simulink library "Library_ASK"  (R2018b)
settings: Solver=VariableStepAuto  StartTime=0.0  StopTime=10.0  RelTol=1e-3  EnableMultiTasking=on
undefined symbols (not defined in the file): akt_2GTR_az_HA, akt_2GTR_az_VA, akt_2GTR_rn_HA, akt_2GTR_rn_VA, akt_GTR_az_HA, akt_GTR_az_VA, akt_GTR_rn_HA, akt_GTR_rn_VA, alpha, b_zahn, beta_b, breakpointset, choose_ulg, DiscIntNeverNeededParam, eps_1, eps_2, eps_alpha, eta_aa, eta_Kegel_max, Fx_LSD_max, Fx_mUELG_max, i_DF, i_Kegelrad_OD, i_TRM_G1_HA, i_TRM_G1_VA, i_TRM_G2_HA, i_TRM_G2_VA, i_TRM_HA, i_TRM_Stufe_1_HA, i_TRM_Stufe_1_VA, i_TRM_Stufe_2_HA, i_TRM_Stufe_2_VA, i_TRM_VA, M_Cl_LSD_max, M_Cl_mUELG_max, M_EM_max, M_Kupplung_mUELG_Schlepp, mu_cl_LSD, mu_cl_mUELG, n_EM_max, n_Stufen_TRM_HA, n_Stufen_TRM_VA, ndyn_oil, nreib_LSD, nreib_mUELG, par_MDT, par_VEH, Ra, rm_LSD, rm_mUELG, select_Traktion_split, stepsize, wkg_Diff_mUELG, wkg_GTR, X_L, z_atts, z_ayc, z_ayc_lr, z_ayc_rl
libraries: simulink x23, $bdroot x6
(part 3 of 4)

== system Library_ASK/Mehrstufiges und mehrgängiges Getriebe/Subsystem ==
  WKG : Inport
  Inputleistung : Inport  Port=2
  Abs : Abs
  Add : Sum  Inputs=+-
  Constant : Constant
  Product5 : Product
  "W -> kW" : Gain  Gain=0.001
  Verlustleistung [kW] : Outport
  wires:
  Constant/1 -> Add/1
  Inputleistung/1 -> Product5/2
  Add/1 -> Product5/1
  Abs/1 -> "W -> kW"/1
  Product5/1 -> Abs/1
  "W -> kW"/1 -> Verlustleistung [kW]/1
  WKG/1 -> Add/2

== system Library_ASK/Momentenrückführung az HA/Fall Eingängiges Getriebe ==
  Radwunschmoment : Inport
  eta_HA : Inport  Port=2
  Enable : EnablePort
  Constant : Constant  Value=i_TRM_HA
  Divide2 : Product  Inputs=*//
  Motorwunschmoment : Outport
  wires:
  Radwunschmoment/1 -> Divide2/1
  Constant/1 -> Divide2/2
  Divide2/1 -> Motorwunschmoment/1
  eta_HA/1 -> Divide2/3

== system Library_ASK/Momentenrückführung az HA/Fall zweigängiges Getriebe ==
  note: auf diese Weise wird die Goto/From - Rückführung aus dem EM -Block überflüssig
  Radwunschmoment : Inport
  Mittlere Raddrehzahl : Inport  Port=2
  eta_HA : Inport  Port=3
  Enable : EnablePort
  Constant : Constant  Value=i_TRM_G1_HA
  Constant1 : Constant  Value=i_TRM_G2_HA
  Constant2 : Constant  Value=n_EM_max
  Divide1 : Product  Inputs=*//
  MATLAB Function : MATLAB Function  TreatAsAtomicUnit=on
  Product : Product
  Motorwunschmoment : Outport
  wires:
  Product/1 -> MATLAB Function/1(n_EM)
  Mittlere Raddrehzahl/1 -> Product/1
  Divide1/1 -> Motorwunschmoment/1
  Constant/1 -> MATLAB Function/3(i_TRM_G1), Product/2
  Radwunschmoment/1 -> Divide1/1
  MATLAB Function/1(i_TRM) -> Divide1/2
  Constant1/1 -> MATLAB Function/4(i_TRM_G2)
  Constant2/1 -> MATLAB Function/2(n_EM_max)
  eta_HA/1 -> Divide1/3

== system Library_ASK/Momentenrückführung az VA/Fall Eingängiges Getriebe ==
  Radwunschmoment : Inport
  eta_VA : Inport  Port=2
  Enable : EnablePort
  Constant : Constant  Value=i_TRM_VA
  Divide2 : Product  Inputs=*//
  Motorwunschmoment : Outport
  wires:
  Divide2/1 -> Motorwunschmoment/1
  Constant/1 -> Divide2/2
  Radwunschmoment/1 -> Divide2/1
  eta_VA/1 -> Divide2/3

== system Library_ASK/Momentenrückführung az VA/Fall zweigängiges Getriebe ==
  note: auf diese Weise wird die Goto/From - Rückführung aus dem EM -Block überflüssig
  Radwunschmoment : Inport
  Mittlere Raddrehzahl : Inport  Port=2
  eta_VA : Inport  Port=3
  Enable : EnablePort
  Constant : Constant  Value=i_TRM_G1_VA
  Constant1 : Constant  Value=i_TRM_G2_VA
  Constant2 : Constant  Value=n_EM_max
  Divide1 : Product  Inputs=*//
  MATLAB Function : MATLAB Function  TreatAsAtomicUnit=on
  Product : Product
  Motorwunschmoment : Outport
  wires:
  Constant2/1 -> MATLAB Function/2(n_EM_max)
  Constant1/1 -> MATLAB Function/4(i_TRM_G2)
  MATLAB Function/1(i_TRM) -> Divide1/2
  Radwunschmoment/1 -> Divide1/1
  Constant/1 -> Product/2, MATLAB Function/3(i_TRM_G1)
  Divide1/1 -> Motorwunschmoment/1
  Mittlere Raddrehzahl/1 -> Product/1
  Product/1 -> MATLAB Function/1(n_EM)
  eta_VA/1 -> Divide1/3

== system Library_ASK/Momentenrückführung rn HA/Fall Eingängiges Getriebe ==
  Radwunschmoment : Inport
  eta_HA : Inport  Port=2
  Enable : EnablePort
  Constant : Constant  Value=i_TRM_HA
  Divide2 : Product  Inputs=*//
  Motorwunschmoment : Outport
  wires:
  Divide2/1 -> Motorwunschmoment/1
  Constant/1 -> Divide2/2
  Radwunschmoment/1 -> Divide2/1
  eta_HA/1 -> Divide2/3

== system Library_ASK/Momentenrückführung rn HA/Fall zweigängiges Getriebe ==
  note: auf diese Weise wird die Goto/From - Rückführung aus dem EM -Block überflüssig
  Radwunschmoment : Inport
  Raddrehzahl : Inport  Port=2
  eta_HA : Inport  Port=3
  Enable : EnablePort
  Constant : Constant  Value=i_TRM_G1_HA
  Constant1 : Constant  Value=i_TRM_G2_HA
  Constant2 : Constant  Value=n_EM_max
  Demux : Demux  Outputs=2
  Divide1 : Product  Inputs=*//
  MATLAB Function : MATLAB Function  TreatAsAtomicUnit=on
  MATLAB Function1 : MATLAB Function  TreatAsAtomicUnit=on
  Mux : Mux  Inputs=2
  Product : Product
  Motorwunschmoment : Outport
  wires:
  MATLAB Function1/1(i_TRM) -> Mux/2
  MATLAB Function/1(i_TRM) -> Mux/1
  Mux/1 -> Divide1/2
  Demux/2 -> MATLAB Function1/1(n_EM)  "Linkes Rad"
  Demux/1 -> MATLAB Function/1(n_EM)  "Rechtes Rad"
  Constant2/1 -> MATLAB Function/2(n_EM_max), MATLAB Function1/2(n_EM_max)
  Constant1/1 -> MATLAB Function/4(i_TRM_G2), MATLAB Function1/4(i_TRM_G2)
  Radwunschmoment/1 -> Divide1/1
  Constant/1 -> Product/2, MATLAB Function/3(i_TRM_G1), MATLAB Function1/3(i_TRM_G1)
  Divide1/1 -> Motorwunschmoment/1
  Raddrehzahl/1 -> Product/1
  Product/1 -> Demux/1
  eta_HA/1 -> Divide1/3

== system Library_ASK/Momentenrückführung rn VA/Fall Eingängiges Getriebe ==
  Radwunschmoment : Inport
  eta_VA : Inport  Port=2
  Enable : EnablePort
  Constant : Constant  Value=i_TRM_VA
  Divide2 : Product  Inputs=*//
  Motorwunschmoment : Outport
  wires:
  Radwunschmoment/1 -> Divide2/1
  Constant/1 -> Divide2/2
  Divide2/1 -> Motorwunschmoment/1
  eta_VA/1 -> Divide2/3

== system Library_ASK/Momentenrückführung rn VA/Fall zweigängiges Getriebe ==
  note: auf diese Weise wird die Goto/From - Rückführung aus dem EM -Block überflüssig
  Radwunschmoment : Inport
  Raddrehzahl : Inport  Port=2
  eta_VA : Inport  Port=3
  Enable : EnablePort
  Constant : Constant  Value=i_TRM_G1_VA
  Constant1 : Constant  Value=i_TRM_G2_VA
  Constant2 : Constant  Value=n_EM_max
  Demux : Demux  Outputs=2
  Divide1 : Product  Inputs=*//
  MATLAB Function : MATLAB Function  TreatAsAtomicUnit=on
  MATLAB Function1 : MATLAB Function  TreatAsAtomicUnit=on
  Mux : Mux  Inputs=2
  Product : Product
  Motorwunschmoment : Outport
  wires:
  Product/1 -> Demux/1
  Raddrehzahl/1 -> Product/1
  Divide1/1 -> Motorwunschmoment/1
  Constant/1 -> MATLAB Function1/3(i_TRM_G1), MATLAB Function/3(i_TRM_G1), Product/2
  Radwunschmoment/1 -> Divide1/1
  Constant1/1 -> MATLAB Function1/4(i_TRM_G2), MATLAB Function/4(i_TRM_G2)
  Constant2/1 -> MATLAB Function1/2(n_EM_max), MATLAB Function/2(n_EM_max)
  Demux/1 -> MATLAB Function/1(n_EM)  "Rechtes Rad"
  Demux/2 -> MATLAB Function1/1(n_EM)  "Linkes Rad"
  Mux/1 -> Divide1/2
  MATLAB Function/1(i_TRM) -> Mux/1
  MATLAB Function1/1(i_TRM) -> Mux/2
  eta_VA/1 -> Divide1/3

== system Library_ASK/NWH Planetengetriebe/Berechnung Hv ==
  note: wegen Hohlrad
  z_Ritzel : Inport
  z_Rad : Inport  Port=2
  Abs : Abs
  Add : Sum
  Add1 : Sum  Inputs=+-++
  Berechnung i : Product  Inputs=*/
  Constant : Constant
  Constant1 : Constant
  Divide : Product  Inputs=*///
  Gain : Gain  Gain=pi
  Grundkreisschrägungswinkel : Constant  Value=beta_b
  Kopfüberdeckung Rad : Constant  Value=eps_2
  Kopfüberdeckung Ritzel : Constant  Value=eps_1
  Math Function : Math  Operator=square  SaturateOnIntegerOverflow=on
  Math Function1 : Math  Operator=square  SaturateOnIntegerOverflow=on
  Product : Product
  Profilüberdeckung : Constant  Value=eps_alpha
  Trigonometric Function : Trigonometry  Operator=cos
  Hv : Outport
  wires:
  z_Ritzel/1 -> Divide/3, Berechnung i/2
  z_Rad/1 -> Abs/1
  Constant1/1 -> Add/1
  Berechnung i/1 -> Divide/2, Add/2
  Add/1 -> Gain/1
  Grundkreisschrägungswinkel/1 -> Trigonometric Function/1
  Gain/1 -> Divide/1
  Trigonometric Function/1 -> Divide/4
  Divide/1 -> Product/1
  Kopfüberdeckung Ritzel/1 -> Math Function/1
  Math Function/1 -> Add1/3
  Math Function1/1 -> Add1/4
  Kopfüberdeckung Rad/1 -> Math Function1/1
  Profilüberdeckung/1 -> Add1/2
  Constant/1 -> Add1/1
  Add1/1 -> Product/2
  Product/1 -> Hv/1
  Abs/1 -> Berechnung i/1

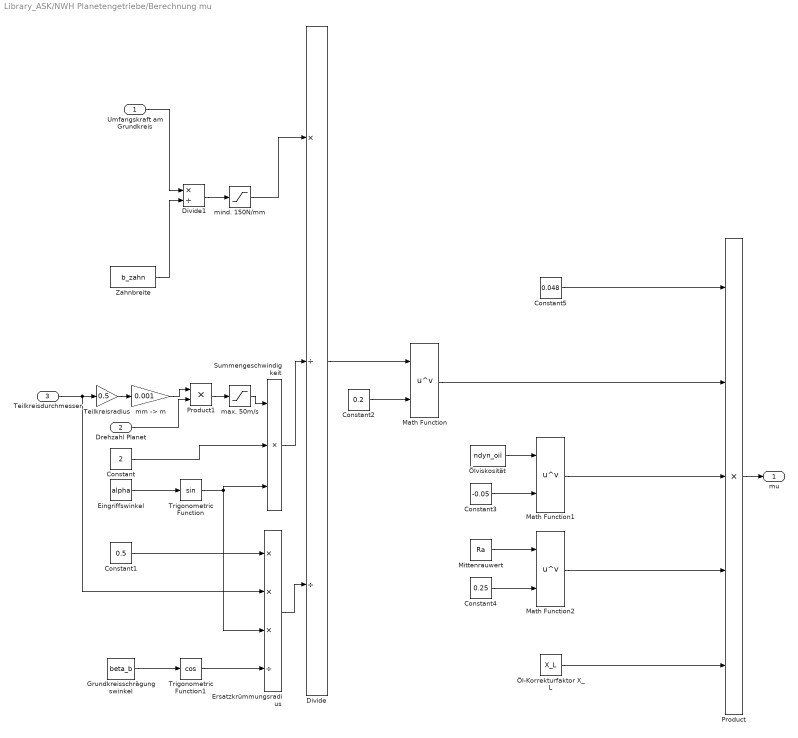
== system Library_ASK/NWH Planetengetriebe/Berechnung mu ==
  Umfangskraft am Grundkreis : Inport
  Drehzahl Planet : Inport  Port=2
  Teilkreisdurchmesser : Inport  Port=3
  Constant : Constant  Value=2
  Constant1 : Constant  Value=0.5
  Constant2 : Constant  Value=0.2
  Constant3 : Constant  Value=-0.05
  Constant4 : Constant  Value=0.25
  Constant5 : Constant  Value=0.048
  Divide : Product  Inputs=*//
  Divide1 : Product  Inputs=*/
  Eingriffswinkel : Constant  Value=alpha
  Ersatzkrümmungsradius : Product  Inputs=***/
  Grundkreisschrägungswinkel : Constant  Value=beta_b
  Math Function : Math  Operator=pow  SaturateOnIntegerOverflow=on
  Math Function1 : Math  Operator=pow  SaturateOnIntegerOverflow=on
  Math Function2 : Math  Operator=pow  SaturateOnIntegerOverflow=on
  Mittenrauwert : Constant  Value=Ra
  Product : Product  Inputs=5
  Product1 : Product
  Summengeschwindigkeit : Product  Inputs=3
  Teilkreisradius : Gain  Gain=0.5
  Trigonometric Function : Trigonometry
  Trigonometric Function1 : Trigonometry  Operator=cos
  Zahnbreite : Constant  Value=b_zahn
  max. 50m/s : Saturate  UpperLimit=50  LowerLimit=0
  mind. 150N/mm : Saturate  UpperLimit=inf  LowerLimit=150
  "mm -> m" : Gain  Gain=0.001
  Öl-Korrekturfaktor X_L : Constant  Value=X_L
  Ölviskosität : Constant  Value=ndyn_oil
  mu : Outport
  wires:
  Zahnbreite/1 -> Divide1/2
  Teilkreisdurchmesser/1 -> Teilkreisradius/1, Ersatzkrümmungsradius/2
  Teilkreisradius/1 -> "mm -> m"/1
  Drehzahl Planet/1 -> Product1/2
  Constant/1 -> Summengeschwindigkeit/2
  Trigonometric Function/1 -> Summengeschwindigkeit/3, Ersatzkrümmungsradius/3
  Eingriffswinkel/1 -> Trigonometric Function/1
  Summengeschwindigkeit/1 -> Divide/2
  Constant1/1 -> Ersatzkrümmungsradius/1
  Trigonometric Function1/1 -> Ersatzkrümmungsradius/4
  Grundkreisschrägungswinkel/1 -> Trigonometric Function1/1
  Ersatzkrümmungsradius/1 -> Divide/3
  Constant2/1 -> Math Function/2
  Divide/1 -> Math Function/1
  Constant3/1 -> Math Function1/2
  Ölviskosität/1 -> Math Function1/1
  Mittenrauwert/1 -> Math Function2/1
  Constant4/1 -> Math Function2/2
  Constant5/1 -> Product/1
  Math Function/1 -> Product/2
  Math Function1/1 -> Product/3
  Math Function2/1 -> Product/4
  Öl-Korrekturfaktor X_L/1 -> Product/5
  Product/1 -> mu/1
  Umfangskraft am Grundkreis/1 -> Divide1/1
  "mm -> m"/1 -> Product1/1
  Divide1/1 -> mind. 150N/mm/1
  mind. 150N/mm/1 -> Divide/1
  Product1/1 -> max. 50m/s/1
  max. 50m/s/1 -> Summengeschwindigkeit/1

== system Library_ASK/NWH Stufengetriebe/Berechnung Hv ==
  note: wegen Hohlrad
  z_Ritzel : Inport
  z_Rad : Inport  Port=2
  Abs : Abs
  Add : Sum
  Add1 : Sum  Inputs=+-++
  Berechnung i : Product  Inputs=*/
  Constant : Constant
  Constant1 : Constant
  Divide : Product  Inputs=*///
  Gain : Gain  Gain=pi
  Grundkreisschrägungswinkel : Constant  Value=beta_b
  Kopfüberdeckung Rad : Constant  Value=eps_2
  Kopfüberdeckung Ritzel : Constant  Value=eps_1
  Math Function : Math  Operator=square  SaturateOnIntegerOverflow=on
  Math Function1 : Math  Operator=square  SaturateOnIntegerOverflow=on
  Product : Product
  Profilüberdeckung : Constant  Value=eps_alpha
  Trigonometric Function : Trigonometry  Operator=cos
  Hv : Outport
  wires:
  Abs/1 -> Berechnung i/1
  Product/1 -> Hv/1
  Add1/1 -> Product/2
  Constant/1 -> Add1/1
  Profilüberdeckung/1 -> Add1/2
  Kopfüberdeckung Rad/1 -> Math Function1/1
  Math Function1/1 -> Add1/4
  Math Function/1 -> Add1/3
  Kopfüberdeckung Ritzel/1 -> Math Function/1
  Divide/1 -> Product/1
  Trigonometric Function/1 -> Divide/4
  Gain/1 -> Divide/1
  Grundkreisschrägungswinkel/1 -> Trigonometric Function/1
  Add/1 -> Gain/1
  Berechnung i/1 -> Add/2, Divide/2
  Constant1/1 -> Add/1
  z_Rad/1 -> Abs/1
  z_Ritzel/1 -> Berechnung i/2, Divide/3

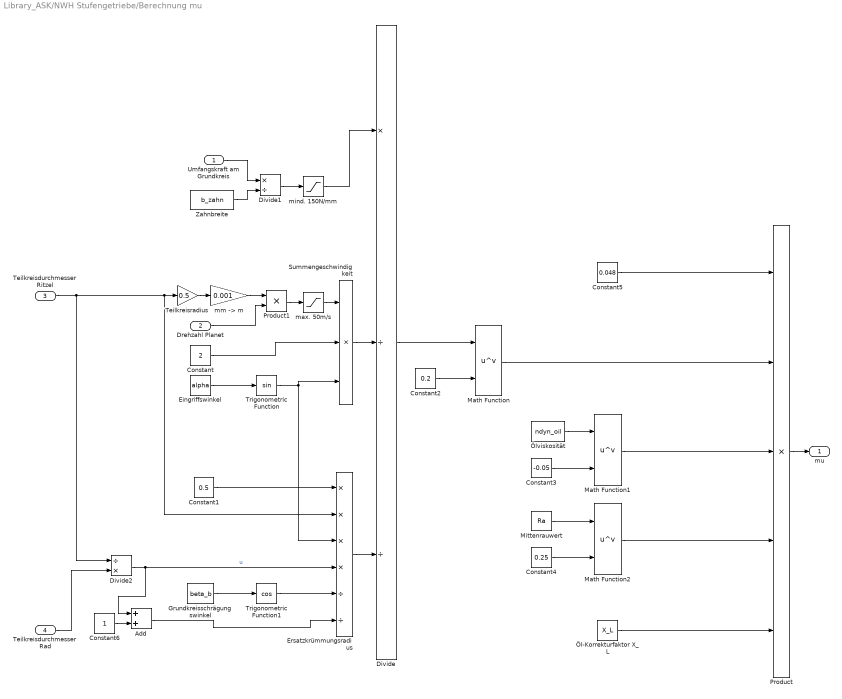
== system Library_ASK/NWH Stufengetriebe/Berechnung mu ==
  Umfangskraft am Grundkreis : Inport
  Drehzahl Planet : Inport  Port=2
  Teilkreisdurchmesser Ritzel : Inport  Port=3
  Teilkreisdurchmesser Rad : Inport  Port=4
  Add : Sum
  Constant : Constant  Value=2
  Constant1 : Constant  Value=0.5
  Constant2 : Constant  Value=0.2
  Constant3 : Constant  Value=-0.05
  Constant4 : Constant  Value=0.25
  Constant5 : Constant  Value=0.048
  Constant6 : Constant
  Divide : Product  Inputs=*//
  Divide1 : Product  Inputs=*/
  Divide2 : Product  Inputs=/*
  Eingriffswinkel : Constant  Value=alpha
  Ersatzkrümmungsradius : Product  Inputs=****//
  Grundkreisschrägungswinkel : Constant  Value=beta_b
  Math Function : Math  Operator=pow  SaturateOnIntegerOverflow=on
  Math Function1 : Math  Operator=pow  SaturateOnIntegerOverflow=on
  Math Function2 : Math  Operator=pow  SaturateOnIntegerOverflow=on
  Mittenrauwert : Constant  Value=Ra
  Product : Product  Inputs=5
  Product1 : Product
  Summengeschwindigkeit : Product  Inputs=3
  Teilkreisradius : Gain  Gain=0.5
  Trigonometric Function : Trigonometry
  Trigonometric Function1 : Trigonometry  Operator=cos
  Zahnbreite : Constant  Value=b_zahn
  max. 50m/s : Saturate  UpperLimit=50  LowerLimit=1
  mind. 150N/mm : Saturate  UpperLimit=inf  LowerLimit=150
  "mm -> m" : Gain  Gain=0.001
  Öl-Korrekturfaktor X_L : Constant  Value=X_L
  Ölviskosität : Constant  Value=ndyn_oil
  mu : Outport
  wires:
  max. 50m/s/1 -> Summengeschwindigkeit/1
  Product1/1 -> max. 50m/s/1
  mind. 150N/mm/1 -> Divide/1
  Divide1/1 -> mind. 150N/mm/1
  "mm -> m"/1 -> Product1/1
  Umfangskraft am Grundkreis/1 -> Divide1/1
  Product/1 -> mu/1
  Öl-Korrekturfaktor X_L/1 -> Product/5
  Math Function2/1 -> Product/4
  Math Function1/1 -> Product/3
  Math Function/1 -> Product/2
  Constant5/1 -> Product/1
  Constant4/1 -> Math Function2/2
  Mittenrauwert/1 -> Math Function2/1
  Ölviskosität/1 -> Math Function1/1
  Constant3/1 -> Math Function1/2
  Divide/1 -> Math Function/1
  Constant2/1 -> Math Function/2
  Ersatzkrümmungsradius/1 -> Divide/3
  Grundkreisschrägungswinkel/1 -> Trigonometric Function1/1
  Trigonometric Function1/1 -> Ersatzkrümmungsradius/5
  Constant1/1 -> Ersatzkrümmungsradius/1
  Summengeschwindigkeit/1 -> Divide/2
  Eingriffswinkel/1 -> Trigonometric Function/1
  Trigonometric Function/1 -> Ersatzkrümmungsradius/3, Summengeschwindigkeit/3
  Constant/1 -> Summengeschwindigkeit/2
  Drehzahl Planet/1 -> Product1/2
  Teilkreisradius/1 -> "mm -> m"/1
  Teilkreisdurchmesser Ritzel/1 -> Divide2/1, Ersatzkrümmungsradius/2, Teilkreisradius/1
  Zahnbreite/1 -> Divide1/2
  Teilkreisdurchmesser Rad/1 -> Divide2/2
  Divide2/1 -> Add/1, Ersatzkrümmungsradius/4  "u"
  Add/1 -> Ersatzkrümmungsradius/6
  Constant6/1 -> Add/2

== system Library_ASK/Simple E-Maschine/Subsystem ==
  Drehzahl : Inport
  Stellmoment : Inport  Port=2
  WKG : Inport  Port=3
  Vorzeidchen Antriebsmoment : Inport  Port=4
  1-WKG : Inport  Port=5
  Abs : Abs
  Math Function : Math  Operator=pow  SaturateOnIntegerOverflow=on
  MinMax : MinMax  Function=max  Inputs=2
  Product1 : Product  Inputs=***
  Product2 : Product  Inputs=**
  Product3 : Product  Inputs=**
  "W -> kW1" : Gain  Gain=-1
  Verlustleistung : Outport
  Leistungsaufnahme : Outport  Port=2  InitialOutput=0
  wires:
  Product2/1 -> Verlustleistung/1
  1-WKG/1 -> Product2/2
  Stellmoment/1 -> Product3/2, Product1/2
  Product1/1 -> MinMax/1, Leistungsaufnahme/1
  Math Function/1 -> Product1/3
  "W -> kW1"/1 -> Math Function/2
  Vorzeidchen Antriebsmoment/1 -> "W -> kW1"/1
  Drehzahl/1 -> Product3/1, Product1/1
  WKG/1 -> Math Function/1
  MinMax/1 -> Product2/1
  Product3/1 -> Abs/1
  Abs/1 -> MinMax/2

== system Library_ASK/Simple E-Maschine/generatorischer WKG ==
  Drehzahl : Inport
  Moment : Inport  Port=2
  Enable : EnablePort
  Abs : Abs
  Add : Sum  Inputs=+-
  Constant : Constant
  Saturation : Saturate  UpperLimit=1  LowerLimit=0.05
  Saturation2 : Saturate  UpperLimit=1  LowerLimit=0.2
  Switch : Switch  Criteria=u2 > Threshold  Threshold=120
  Wirkungsgradkennfeld nach Pesce Generatorbetrieb : Lookup_n-D  BreakpointsForDimension1=Gen_Pesce_y  BreakpointsForDimension2=Gen_Pesce_z  Table=Gen_Pesce_Mat  UseLastTableValue=on  InternalRulePriority=Speed  RndMeth=Simplest  InputSameDT=on
  WKG : Outport
  1-WKG : Outport  Port=2
  wires:
  Abs/1 -> Wirkungsgradkennfeld nach Pesce Generatorbetrieb/2
  Add/1 -> 1-WKG/1
  Constant/1 -> Add/1
  Wirkungsgradkennfeld nach Pesce Generatorbetrieb/1 -> Saturation2/1, Saturation/1
  Moment/1 -> Abs/1
  Switch/1 -> WKG/1, Add/2
  Drehzahl/1 -> Switch/2, Wirkungsgradkennfeld nach Pesce Generatorbetrieb/1
  Saturation/1 -> Switch/1
  Saturation2/1 -> Switch/3

== system Library_ASK/Simple E-Maschine/motorischer WKG ==
  Drehzahl : Inport
  Moment : Inport  Port=2
  Enable : EnablePort
  Add : Sum  Inputs=+-
  Constant : Constant
  Saturation : Saturate  UpperLimit=1  LowerLimit=0.05
  Saturation1 : Saturate  UpperLimit=1  LowerLimit=0.2
  Switch : Switch  Criteria=u2 > Threshold  Threshold=120
  Wirkungsgradkennfeld nach Pesce Motorbetrieb : Lookup_n-D  BreakpointsForDimension1=Mot_Pesce_y  BreakpointsForDimension2=Mot_Pesce_z  Table=Mot_Pesce_Mat  UseLastTableValue=on  InternalRulePriority=Speed  RndMeth=Simplest  InputSameDT=on
  WKG : Outport
  1-WKG : Outport  Port=2
  wires:
  Add/1 -> 1-WKG/1
  Constant/1 -> Add/1
  Wirkungsgradkennfeld nach Pesce Motorbetrieb/1 -> Saturation1/1, Saturation/1
  Moment/1 -> Wirkungsgradkennfeld nach Pesce Motorbetrieb/2
  Drehzahl/1 -> Switch/2, Wirkungsgradkennfeld nach Pesce Motorbetrieb/1
  Switch/1 -> Add/2, WKG/1
  Saturation/1 -> Switch/1
  Saturation1/1 -> Switch/3

== system Library_ASK/Simple E-Maschine radnah/WKG Maschine Links ==
  Moment : Inport
  Drehzahl : Inport  Port=2
  Add1 : Sum
  Constant1 : Constant
  Gain1 : Gain  Gain=0.001
  Logical Operator : Logic  Operator=NOT  AllPortsSameDT=off  OutDataTypeStr=boolean
  Sign : Signum
  Subsystem : $bdroot/Simple E-Maschine/Subsystem  SystemSampleTime=-1
  Switch : Switch  Criteria=u2 > Threshold
  Switch1 : Switch  Criteria=u2 > Threshold
  generatorischer WKG : Subsystem
  motorischer WKG : Subsystem
  WKG links : Outport
  Verlustleistung links : Outport  Port=2
  Leistungsaufnahme links : Outport  Port=3
  wires:
  Gain1/1 -> Verlustleistung links/1
  Subsystem/2 -> Leistungsaufnahme links/1
  Subsystem/1 -> Gain1/1
  Switch/1 -> WKG links/1, Subsystem/3
  Switch1/1 -> Subsystem/5
  Logical Operator/1 -> generatorischer WKG/Enable
  motorischer WKG/1(WKG) -> Switch/1
  Constant1/1 -> Add1/2
  Sign/1 -> Add1/1, Subsystem/4
  Add1/1 -> Logical Operator/1, Switch/2, Switch1/2, motorischer WKG/Enable
  motorischer WKG/2(1-WKG) -> Switch1/1
  generatorischer WKG/1(WKG) -> Switch/3
  Drehzahl/1 -> generatorischer WKG/1(Drehzahl), motorischer WKG/1(Drehzahl), Subsystem/1
  Moment/1 -> generatorischer WKG/2(Moment), motorischer WKG/2(Moment), Sign/1, Subsystem/2
  generatorischer WKG/2(1-WKG) -> Switch1/3

== system Library_ASK/Simple E-Maschine radnah/WKG Maschine Rechts ==
  Moment : Inport
  Drehzahl : Inport  Port=2
  Add1 : Sum
  Constant1 : Constant
  Gain1 : Gain  Gain=0.001
  Logical Operator : Logic  Operator=NOT  AllPortsSameDT=off  OutDataTypeStr=boolean
  Sign : Signum
  Subsystem : $bdroot/Simple E-Maschine/Subsystem  SystemSampleTime=-1
  Switch : Switch  Criteria=u2 > Threshold
  Switch1 : Switch  Criteria=u2 > Threshold
  generatorischer WKG : Subsystem
  motorischer WKG : Subsystem
  WKG rechts : Outport
  Verlustleistung rechts : Outport  Port=2
  Leistungsaufnahme rechts : Outport  Port=3
  wires:
  Gain1/1 -> Verlustleistung rechts/1
  Sign/1 -> Add1/1, Subsystem/4
  Moment/1 -> Sign/1, motorischer WKG/2(Moment), generatorischer WKG/2(Moment), Subsystem/2
  Switch1/1 -> Subsystem/5
  Subsystem/1 -> Gain1/1
  Switch/1 -> WKG rechts/1, Subsystem/3
  Subsystem/2 -> Leistungsaufnahme rechts/1
  Drehzahl/1 -> motorischer WKG/1(Drehzahl), generatorischer WKG/1(Drehzahl), Subsystem/1
  generatorischer WKG/2(1-WKG) -> Switch1/3
  generatorischer WKG/1(WKG) -> Switch/3
  motorischer WKG/2(1-WKG) -> Switch1/1
  Add1/1 -> motorischer WKG/Enable, Switch1/2, Switch/2, Logical Operator/1
  Constant1/1 -> Add1/2
  motorischer WKG/1(WKG) -> Switch/1
  Logical Operator/1 -> generatorischer WKG/Enable

== system Library_ASK/Simple E-Maschine radnah ALT/WKG Maschine Links ==
  Moment : Inport
  Drehzahl : Inport  Port=2
  Add1 : Sum
  Constant1 : Constant
  Gain1 : Gain  Gain=0.001
  Logical Operator : Logic  Operator=NOT  AllPortsSameDT=off  OutDataTypeStr=boolean
  Sign : Signum
  Subsystem : $bdroot/Simple E-Maschine/Subsystem  SystemSampleTime=-1
  Switch : Switch  Criteria=u2 > Threshold
  Switch1 : Switch  Criteria=u2 > Threshold
  generatorischer WKG : Subsystem
  motorischer WKG : Subsystem
  WKG links : Outport
  Verlustleistung links : Outport  Port=2
  Leistungsaufnahme links : Outport  Port=3
  wires:
  generatorischer WKG/2(1-WKG) -> Switch1/3
  Moment/1 -> Subsystem/2, Sign/1, motorischer WKG/2(Moment), generatorischer WKG/2(Moment)
  Drehzahl/1 -> Subsystem/1, motorischer WKG/1(Drehzahl), generatorischer WKG/1(Drehzahl)
  generatorischer WKG/1(WKG) -> Switch/3
  motorischer WKG/2(1-WKG) -> Switch1/1
  Add1/1 -> motorischer WKG/Enable, Switch1/2, Switch/2, Logical Operator/1
  Sign/1 -> Subsystem/4, Add1/1
  Constant1/1 -> Add1/2
  motorischer WKG/1(WKG) -> Switch/1
  Logical Operator/1 -> generatorischer WKG/Enable
  Switch1/1 -> Subsystem/5
  Switch/1 -> Subsystem/3, WKG links/1
  Subsystem/1 -> Gain1/1
  Subsystem/2 -> Leistungsaufnahme links/1
  Gain1/1 -> Verlustleistung links/1

== system Library_ASK/Simple E-Maschine radnah ALT/WKG Maschine Rechts ==
  Moment : Inport
  Drehzahl : Inport  Port=2
  Add1 : Sum
  Constant1 : Constant
  Gain1 : Gain  Gain=0.001
  Logical Operator : Logic  Operator=NOT  AllPortsSameDT=off  OutDataTypeStr=boolean
  Sign : Signum
  Subsystem : $bdroot/Simple E-Maschine/Subsystem  SystemSampleTime=-1
  Switch : Switch  Criteria=u2 > Threshold
  Switch1 : Switch  Criteria=u2 > Threshold
  generatorischer WKG : Subsystem
  motorischer WKG : Subsystem
  WKG rechts : Outport
  Verlustleistung rechts : Outport  Port=2
  Leistungsaufnahme rechts : Outport  Port=3
  wires:
  Logical Operator/1 -> generatorischer WKG/Enable
  motorischer WKG/1(WKG) -> Switch/1
  Constant1/1 -> Add1/2
  Add1/1 -> Logical Operator/1, Switch/2, Switch1/2, motorischer WKG/Enable
  motorischer WKG/2(1-WKG) -> Switch1/1
  generatorischer WKG/1(WKG) -> Switch/3
  generatorischer WKG/2(1-WKG) -> Switch1/3
  Drehzahl/1 -> Subsystem/1, generatorischer WKG/1(Drehzahl), motorischer WKG/1(Drehzahl)
  Subsystem/2 -> Leistungsaufnahme rechts/1
  Switch/1 -> Subsystem/3, WKG rechts/1
  Subsystem/1 -> Gain1/1
  Switch1/1 -> Subsystem/5
  Moment/1 -> Subsystem/2, generatorischer WKG/2(Moment), motorischer WKG/2(Moment), Sign/1
  Sign/1 -> Subsystem/4, Add1/1
  Gain1/1 -> Verlustleistung rechts/1

== system Library_ASK/Zweigängiges Getriebe az HA/Subsystem ==
  WKG : Inport
  Inputleistung : Inport  Port=2
  Abs : Abs
  Add : Sum  Inputs=+-
  Constant : Constant
  Discrete-Time Integrator : DiscreteIntegrator  gainval=1  SampleTime=-1  ICPrevOutput=DiscIntNeverNeededParam  ICPrevScaledInput=DiscIntNeverNeededParam
  Product5 : Product
  "W -> kW" : Gain  Gain=0.001
  "Ws -> kWh" : Gain  Gain=1/3600000
  Energieverlust [kWh] : Outport
  Verlustleistung [kW] : Outport  Port=2
  wires:
  WKG/1 -> Add/2
  "W -> kW"/1 -> Verlustleistung [kW]/1
  Product5/1 -> Abs/1
  Abs/1 -> Discrete-Time Integrator/1, "W -> kW"/1
  "Ws -> kWh"/1 -> Energieverlust [kWh]/1
  Discrete-Time Integrator/1 -> "Ws -> kWh"/1
  Add/1 -> Product5/1
  Inputleistung/1 -> Product5/2
  Constant/1 -> Add/1

== system Library_ASK/Zweigängiges Getriebe az HA/WKG ==
  note: maximaler Wert im Table im init_MVS auf eta_aa festgelegt
  note: mitlaufender zweiter Gang
  Stufenübersetzung : Inport
  Stufenanzahl : Inport  Port=2
  Eingangsdrehzahl : Inport  Port=3
  Last : Inport  Port=4
  1-D Lookup Table Stufe 1 : Lookup_n-D  NumberOfTableDimensions=1  BreakpointsForDimension1=breakpointset  Table=wkg_GTR  InternalRulePriority=Speed  RndMeth=Simplest  InputSameDT=on
  Constant : Constant  Value=eta_aa
  Math Function : Math  Operator=pow  SaturateOnIntegerOverflow=on
  Product : Product
  Terminator : Terminator
  Terminator1 : Terminator
  Terminator2 : Terminator
  WKG : Outport
  wires:
  Constant/1 -> Product/2
  Product/1 -> WKG/1
  Last/1 -> 1-D Lookup Table Stufe 1/1
  Stufenübersetzung/1 -> Terminator1/1
  Stufenanzahl/1 -> Math Function/2, Terminator2/1
  1-D Lookup Table Stufe 1/1 -> Math Function/1
  Math Function/1 -> Product/1
  Eingangsdrehzahl/1 -> Terminator/1

== system Library_ASK/Zweigängiges Getriebe az VA/Subsystem ==
  WKG : Inport
  Inputleistung : Inport  Port=2
  Abs : Abs
  Add : Sum  Inputs=+-
  Constant : Constant
  Discrete-Time Integrator : DiscreteIntegrator  gainval=1  SampleTime=-1  ICPrevOutput=DiscIntNeverNeededParam  ICPrevScaledInput=DiscIntNeverNeededParam
  Product5 : Product
  "W -> kW" : Gain  Gain=0.001
  "Ws -> kWh" : Gain  Gain=1/3600000
  Energieverlust [kWh] : Outport
  Verlustleistung [kW] : Outport  Port=2
  wires:
  Constant/1 -> Add/1
  Inputleistung/1 -> Product5/2
  Add/1 -> Product5/1
  Discrete-Time Integrator/1 -> "Ws -> kWh"/1
  "Ws -> kWh"/1 -> Energieverlust [kWh]/1
  Abs/1 -> "W -> kW"/1, Discrete-Time Integrator/1
  Product5/1 -> Abs/1
  "W -> kW"/1 -> Verlustleistung [kW]/1
  WKG/1 -> Add/2

== system Library_ASK/Zweigängiges Getriebe az VA/WKG ==
  note: mitlaufender zweiter Gang
  note: maximaler Wert im Table im init_MVS auf eta_aa festgelegt
  Stufenübersetzung : Inport
  Stufenanzahl : Inport  Port=2
  Eingangsdrehzahl : Inport  Port=3
  Last : Inport  Port=4
  1-D Lookup Table Stufe 1 : Lookup_n-D  NumberOfTableDimensions=1  BreakpointsForDimension1=breakpointset  Table=wkg_GTR  InternalRulePriority=Speed  RndMeth=Simplest  InputSameDT=on
  Constant : Constant  Value=eta_aa
  Math Function : Math  Operator=pow  SaturateOnIntegerOverflow=on
  Product : Product
  Terminator : Terminator
  Terminator1 : Terminator
  Terminator2 : Terminator
  WKG : Outport
  wires:
  Eingangsdrehzahl/1 -> Terminator/1
  Math Function/1 -> Product/1
  1-D Lookup Table Stufe 1/1 -> Math Function/1
  Stufenanzahl/1 -> Terminator2/1, Math Function/2
  Stufenübersetzung/1 -> Terminator1/1
  Last/1 -> 1-D Lookup Table Stufe 1/1
  Product/1 -> WKG/1
  Constant/1 -> Product/2

== system Library_ASK/Zweigängiges Getriebe rn HA/Subsystem ==
  WKG : Inport
  Inputleistung : Inport  Port=2
  Abs : Abs
  Add : Sum  Inputs=+-
  Constant : Constant
  Discrete-Time Integrator : DiscreteIntegrator  gainval=1  SampleTime=-1  ICPrevOutput=DiscIntNeverNeededParam  ICPrevScaledInput=DiscIntNeverNeededParam
  Product5 : Product
  "W -> kW" : Gain  Gain=0.001
  "Ws -> kWh" : Gain  Gain=1/3600000
  Energieverlust [kWh] : Outport
  Verlustleistung [kW] : Outport  Port=2
  wires:
  Constant/1 -> Add/1
  Inputleistung/1 -> Product5/2
  Add/1 -> Product5/1
  Discrete-Time Integrator/1 -> "Ws -> kWh"/1
  "Ws -> kWh"/1 -> Energieverlust [kWh]/1
  Abs/1 -> "W -> kW"/1, Discrete-Time Integrator/1
  Product5/1 -> Abs/1
  "W -> kW"/1 -> Verlustleistung [kW]/1
  WKG/1 -> Add/2

== system Library_ASK/Zweigängiges Getriebe rn HA/WKG ==
  note: mitlaufender zweiter Gang
  note: maximaler Wert im Table im init_MVS auf eta_aa festgelegt
  Stufenübersetzung : Inport
  Stufenanzahl : Inport  Port=2
  Eingangsdrehzahl : Inport  Port=3
  Last : Inport  Port=4
  1-D Lookup Table Stufe 1 : Lookup_n-D  NumberOfTableDimensions=1  BreakpointsForDimension1=breakpointset  Table=wkg_GTR  InternalRulePriority=Speed  RndMeth=Simplest  InputSameDT=on
  Constant : Constant  Value=eta_aa
  Math Function : Math  Operator=pow  SaturateOnIntegerOverflow=on
  Product : Product
  Terminator : Terminator
  Terminator1 : Terminator
  Terminator2 : Terminator
  WKG : Outport
  wires:
  Eingangsdrehzahl/1 -> Terminator/1
  Math Function/1 -> Product/1
  1-D Lookup Table Stufe 1/1 -> Math Function/1
  Stufenanzahl/1 -> Terminator2/1, Math Function/2
  Stufenübersetzung/1 -> Terminator1/1
  Last/1 -> 1-D Lookup Table Stufe 1/1
  Product/1 -> WKG/1
  Constant/1 -> Product/2

== system Library_ASK/Zweigängiges Getriebe rn VA/Subsystem ==
  WKG : Inport
  Inputleistung : Inport  Port=2
  Abs : Abs
  Add : Sum  Inputs=+-
  Constant : Constant
  Discrete-Time Integrator : DiscreteIntegrator  gainval=1  SampleTime=-1  ICPrevOutput=DiscIntNeverNeededParam  ICPrevScaledInput=DiscIntNeverNeededParam
  Product5 : Product
  "W -> kW" : Gain  Gain=0.001
  "Ws -> kWh" : Gain  Gain=1/3600000
  Energieverlust [kWh] : Outport
  Verlustleistung [kW] : Outport  Port=2
  wires:
  WKG/1 -> Add/2
  "W -> kW"/1 -> Verlustleistung [kW]/1
  Product5/1 -> Abs/1
  Abs/1 -> Discrete-Time Integrator/1, "W -> kW"/1
  "Ws -> kWh"/1 -> Energieverlust [kWh]/1
  Discrete-Time Integrator/1 -> "Ws -> kWh"/1
  Add/1 -> Product5/1
  Inputleistung/1 -> Product5/2
  Constant/1 -> Add/1

== system Library_ASK/Zweigängiges Getriebe rn VA/WKG ==
  note: maximaler Wert im Table im init_MVS auf eta_aa festgelegt
  note: mitlaufender zweiter Gang
  Stufenübersetzung : Inport
  Stufenanzahl : Inport  Port=2
  Eingangsdrehzahl : Inport  Port=3
  Last : Inport  Port=4
  1-D Lookup Table Stufe 1 : Lookup_n-D  NumberOfTableDimensions=1  BreakpointsForDimension1=breakpointset  Table=wkg_GTR  InternalRulePriority=Speed  RndMeth=Simplest  InputSameDT=on
  Constant : Constant  Value=eta_aa
  Math Function : Math  Operator=pow  SaturateOnIntegerOverflow=on
  Product : Product
  Terminator : Terminator
  Terminator1 : Terminator
  Terminator2 : Terminator
  WKG : Outport
  wires:
  Constant/1 -> Product/2
  Product/1 -> WKG/1
  Last/1 -> 1-D Lookup Table Stufe 1/1
  Stufenübersetzung/1 -> Terminator1/1
  Stufenanzahl/1 -> Math Function/2, Terminator2/1
  1-D Lookup Table Stufe 1/1 -> Math Function/1
  Math Function/1 -> Product/1
  Eingangsdrehzahl/1 -> Terminator/1

== system Library_ASK/mechanisches Ueberlagerungsgetriebe/Kupplung ==
  M_Cl_Wunsch : Inport
  okay : Inport  Port=2
  Constant1 : Constant  Value=0
  Divide1 : Product  Inputs=*/**
  Fx_max : Constant  Value=Fx_mUELG_max
  M-Cl-max : Constant  Value=M_Cl_mUELG_max
  PT1_mUELG : DiscreteTransferFcn  Numerator=[0 9.9950e-04]  Denominator=[1 -0.9990]
  Product : Product  Inputs=4
  Reibflächen : Constant  Value=nreib_mUELG
  Saturation Dynamic : simulink/Discontinuities/Saturation Dynamic  OutMin=[]  OutMax=[]  OutDataTypeStr=Inherit: Same as second input  OutDataType=fixdt(1, 16)  OutScaling=2^-10  DoSatur=off
  Zero-Order Hold2 : ZeroOrderHold  SampleTime=stepsize
  mu_cl : Constant  Value=mu_cl_mUELG
  rm : Constant  Value=rm_mUELG
  M_Kupplung : Outport
  wires:
  M_Cl_Wunsch/1 -> Divide1/1
  Product/1 -> M_Kupplung/1
  okay/1 -> Divide1/4
  Divide1/1 -> Saturation Dynamic/2
  Fx_max/1 -> Divide1/3, Saturation Dynamic/1
  M-Cl-max/1 -> Divide1/2
  rm/1 -> Product/2
  mu_cl/1 -> Product/3
  Reibflächen/1 -> Product/4
  PT1_mUELG/1 -> Product/1
  Constant1/1 -> Saturation Dynamic/3
  Zero-Order Hold2/1 -> PT1_mUELG/1
  Saturation Dynamic/1 -> Zero-Order Hold2/1

== system Library_ASK/mechanisches Ueberlagerungsgetriebe/Lastabhängiger WKG ==
  Eingangsmoment : Inport
  1-D Lookup Table1 : Lookup_n-D  NumberOfTableDimensions=1  BreakpointsForDimension1=breakpointset  Table=wkg_Diff_mUELG  InternalRulePriority=Speed  RndMeth=Simplest  InputSameDT=on
  Abs1 : Abs
  Constant : Constant  Value=M_EM_max
  Constant6 : Constant  Value=i_TRM_VA
  Divide : Product  Inputs=*//
  Saturation2 : Saturate  UpperLimit=1  LowerLimit=0
  WKG : Outport
  wires:
  Eingangsmoment/1 -> Divide/1
  Divide/1 -> Abs1/1
  Constant6/1 -> Divide/3
  1-D Lookup Table1/1 -> WKG/1
  Constant/1 -> Divide/2
  Saturation2/1 -> 1-D Lookup Table1/1
  Abs1/1 -> Saturation2/1

== system Library_ASK/mechanisches Ueberlagerungsgetriebe/Transmission Choice ==
  Wunschmoment rechts1 : Inport
  Wunschmoment links1 : Inport  Port=2
  Constant : Constant  Value=i_DF
  Constant1 : Constant  Value=z_ayc_lr
  Constant2 : Constant  Value=z_atts
  Constant3 : Constant  Value=choose_ulg
  Constant4 : Constant  Value=z_ayc_lr
  MATLAB Function : MATLAB Function  TreatAsAtomicUnit=on
  M_Clutch_Wunsch : Outport
  wires:
  Wunschmoment rechts1/1 -> MATLAB Function/1(M_RW)
  Wunschmoment links1/1 -> MATLAB Function/2(M_LW)
  MATLAB Function/1(M_Clutch) -> M_Clutch_Wunsch/1
  Constant/1 -> MATLAB Function/3(i_DF)
  Constant1/1 -> MATLAB Function/4(z_ayc_lr)
  Constant2/1 -> MATLAB Function/6(z_atts)
  Constant3/1 -> MATLAB Function/7(choose_ulg)
  Constant4/1 -> MATLAB Function/5(z_ayc_rl)

== system Library_ASK/Mehrstufiges Getriebe VA/WKG/Übersetzungsabhängiger Maximalwirkugsgrad ==
  In1 : Inport
  Out1 : Outport
  wires:
  In1/1 -> Out1/1

== system Library_ASK/Simple E-Maschine radnah/WKG Maschine Links/generatorischer WKG ==
  Drehzahl : Inport
  Moment : Inport  Port=2
  Enable : EnablePort
  Abs : Abs
  Add : Sum  Inputs=+-
  Constant : Constant
  Saturation : Saturate  UpperLimit=1  LowerLimit=0.05
  Wirkungsgradkennfeld nach Pesce Generatorbetrieb : Lookup_n-D  BreakpointsForDimension1=Gen_Pesce_y  BreakpointsForDimension2=Gen_Pesce_z  Table=Gen_Pesce_Mat  UseLastTableValue=on  InternalRulePriority=Speed  RndMeth=Simplest  InputSameDT=on
  WKG : Outport
  1-WKG : Outport  Port=2
  wires:
  Saturation/1 -> WKG/1, Add/2
  Abs/1 -> Wirkungsgradkennfeld nach Pesce Generatorbetrieb/2
  Drehzahl/1 -> Wirkungsgradkennfeld nach Pesce Generatorbetrieb/1
  Moment/1 -> Abs/1
  Wirkungsgradkennfeld nach Pesce Generatorbetrieb/1 -> Saturation/1
  Constant/1 -> Add/1
  Add/1 -> 1-WKG/1

== system Library_ASK/Simple E-Maschine radnah/WKG Maschine Links/motorischer WKG ==
  Drehzahl : Inport
  Moment : Inport  Port=2
  Enable : EnablePort
  Add : Sum  Inputs=+-
  Constant : Constant
  Saturation : Saturate  UpperLimit=1  LowerLimit=0.05
  Wirkungsgradkennfeld nach Pesce Motorbetrieb : Lookup_n-D  BreakpointsForDimension1=Mot_Pesce_y  BreakpointsForDimension2=Mot_Pesce_z  Table=Mot_Pesce_Mat  UseLastTableValue=on  InternalRulePriority=Speed  RndMeth=Simplest  InputSameDT=on
  WKG : Outport
  1-WKG : Outport  Port=2
  wires:
  Saturation/1 -> Add/2, WKG/1
  Add/1 -> 1-WKG/1
  Constant/1 -> Add/1
  Wirkungsgradkennfeld nach Pesce Motorbetrieb/1 -> Saturation/1
  Moment/1 -> Wirkungsgradkennfeld nach Pesce Motorbetrieb/2
  Drehzahl/1 -> Wirkungsgradkennfeld nach Pesce Motorbetrieb/1

== system Library_ASK/Simple E-Maschine radnah/WKG Maschine Rechts/generatorischer WKG ==
  Drehzahl : Inport
  Moment : Inport  Port=2
  Enable : EnablePort
  Abs : Abs
  Add : Sum  Inputs=+-
  Constant : Constant
  Saturation : Saturate  UpperLimit=1  LowerLimit=0.05
  Wirkungsgradkennfeld nach Pesce Generatorbetrieb : Lookup_n-D  BreakpointsForDimension1=Gen_Pesce_y  BreakpointsForDimension2=Gen_Pesce_z  Table=Gen_Pesce_Mat  UseLastTableValue=on  InternalRulePriority=Speed  RndMeth=Simplest  InputSameDT=on
  WKG : Outport
  1-WKG : Outport  Port=2
  wires:
  Saturation/1 -> WKG/1, Add/2
  Abs/1 -> Wirkungsgradkennfeld nach Pesce Generatorbetrieb/2
  Drehzahl/1 -> Wirkungsgradkennfeld nach Pesce Generatorbetrieb/1
  Moment/1 -> Abs/1
  Wirkungsgradkennfeld nach Pesce Generatorbetrieb/1 -> Saturation/1
  Constant/1 -> Add/1
  Add/1 -> 1-WKG/1

== system Library_ASK/Simple E-Maschine radnah/WKG Maschine Rechts/motorischer WKG ==
  Drehzahl : Inport
  Moment : Inport  Port=2
  Enable : EnablePort
  Add : Sum  Inputs=+-
  Constant : Constant
  Saturation : Saturate  UpperLimit=1  LowerLimit=0.05
  Wirkungsgradkennfeld nach Pesce Motorbetrieb : Lookup_n-D  BreakpointsForDimension1=Mot_Pesce_y  BreakpointsForDimension2=Mot_Pesce_z  Table=Mot_Pesce_Mat  UseLastTableValue=on  InternalRulePriority=Speed  RndMeth=Simplest  InputSameDT=on
  WKG : Outport
  1-WKG : Outport  Port=2
  wires:
  Saturation/1 -> Add/2, WKG/1
  Add/1 -> 1-WKG/1
  Constant/1 -> Add/1
  Wirkungsgradkennfeld nach Pesce Motorbetrieb/1 -> Saturation/1
  Moment/1 -> Wirkungsgradkennfeld nach Pesce Motorbetrieb/2
  Drehzahl/1 -> Wirkungsgradkennfeld nach Pesce Motorbetrieb/1

== system Library_ASK/Simple E-Maschine radnah ALT/WKG Maschine Links/generatorischer WKG ==
  Drehzahl : Inport
  Moment : Inport  Port=2
  Enable : EnablePort
  Abs : Abs
  Add : Sum  Inputs=+-
  Constant : Constant
  Saturation : Saturate  UpperLimit=1  LowerLimit=0.05
  Wirkungsgradkennfeld nach Pesce Generatorbetrieb : Lookup_n-D  BreakpointsForDimension1=Gen_Pesce_y  BreakpointsForDimension2=Gen_Pesce_z  Table=Gen_Pesce_Mat  UseLastTableValue=on  InternalRulePriority=Speed  RndMeth=Simplest  InputSameDT=on
  WKG : Outport
  1-WKG : Outport  Port=2
  wires:
  Add/1 -> 1-WKG/1
  Constant/1 -> Add/1
  Wirkungsgradkennfeld nach Pesce Generatorbetrieb/1 -> Saturation/1
  Moment/1 -> Abs/1
  Drehzahl/1 -> Wirkungsgradkennfeld nach Pesce Generatorbetrieb/1
  Abs/1 -> Wirkungsgradkennfeld nach Pesce Generatorbetrieb/2
  Saturation/1 -> Add/2, WKG/1

== system Library_ASK/Simple E-Maschine radnah ALT/WKG Maschine Links/motorischer WKG ==
  Drehzahl : Inport
  Moment : Inport  Port=2
  Enable : EnablePort
  Add : Sum  Inputs=+-
  Constant : Constant
  Saturation : Saturate  UpperLimit=1  LowerLimit=0.05
  Wirkungsgradkennfeld nach Pesce Motorbetrieb : Lookup_n-D  BreakpointsForDimension1=Mot_Pesce_y  BreakpointsForDimension2=Mot_Pesce_z  Table=Mot_Pesce_Mat  UseLastTableValue=on  InternalRulePriority=Speed  RndMeth=Simplest  InputSameDT=on
  WKG : Outport
  1-WKG : Outport  Port=2
  wires:
  Drehzahl/1 -> Wirkungsgradkennfeld nach Pesce Motorbetrieb/1
  Moment/1 -> Wirkungsgradkennfeld nach Pesce Motorbetrieb/2
  Wirkungsgradkennfeld nach Pesce Motorbetrieb/1 -> Saturation/1
  Constant/1 -> Add/1
  Add/1 -> 1-WKG/1
  Saturation/1 -> WKG/1, Add/2

== system Library_ASK/Simple E-Maschine radnah ALT/WKG Maschine Rechts/generatorischer WKG ==
  Drehzahl : Inport
  Moment : Inport  Port=2
  Enable : EnablePort
  Abs : Abs
  Add : Sum  Inputs=+-
  Constant : Constant
  Saturation : Saturate  UpperLimit=1  LowerLimit=0.05
  Wirkungsgradkennfeld nach Pesce Generatorbetrieb : Lookup_n-D  BreakpointsForDimension1=Gen_Pesce_y  BreakpointsForDimension2=Gen_Pesce_z  Table=Gen_Pesce_Mat  UseLastTableValue=on  InternalRulePriority=Speed  RndMeth=Simplest  InputSameDT=on
  WKG : Outport
  1-WKG : Outport  Port=2
  wires:
  Add/1 -> 1-WKG/1
  Constant/1 -> Add/1
  Wirkungsgradkennfeld nach Pesce Generatorbetrieb/1 -> Saturation/1
  Moment/1 -> Abs/1
  Drehzahl/1 -> Wirkungsgradkennfeld nach Pesce Generatorbetrieb/1
  Abs/1 -> Wirkungsgradkennfeld nach Pesce Generatorbetrieb/2
  Saturation/1 -> Add/2, WKG/1

== system Library_ASK/Simple E-Maschine radnah ALT/WKG Maschine Rechts/motorischer WKG ==
  Drehzahl : Inport
  Moment : Inport  Port=2
  Enable : EnablePort
  Add : Sum  Inputs=+-
  Constant : Constant
  Saturation : Saturate  UpperLimit=1  LowerLimit=0.05
  Wirkungsgradkennfeld nach Pesce Motorbetrieb : Lookup_n-D  BreakpointsForDimension1=Mot_Pesce_y  BreakpointsForDimension2=Mot_Pesce_z  Table=Mot_Pesce_Mat  UseLastTableValue=on  InternalRulePriority=Speed  RndMeth=Simplest  InputSameDT=on
  WKG : Outport
  1-WKG : Outport  Port=2
  wires:
  Drehzahl/1 -> Wirkungsgradkennfeld nach Pesce Motorbetrieb/1
  Moment/1 -> Wirkungsgradkennfeld nach Pesce Motorbetrieb/2
  Wirkungsgradkennfeld nach Pesce Motorbetrieb/1 -> Saturation/1
  Constant/1 -> Add/1
  Add/1 -> 1-WKG/1
  Saturation/1 -> WKG/1, Add/2

== matlab function Library_ASK/mechanisches Ueberlagerungsgetriebe/MATLAB Function ==
  data: M_Kupplung input; M_Kupplung_mUELG_Schlepp input; okay_CL input; okay_CR input; M_Rad_rechts output; M_ein input; M_RW input; M_LW input; n_ein input; nri input; nli input; eta_Diff_mUELG input; eta_Verz_mUELG input; i_DF input; M_Rad_links output; P_Cl_V output; P_Cl_Schlepp output; P_Verz_V output; z_ayc_lr input; z_ayc_rl input; z_atts input; choose_ulg input
function [M_Rad_rechts, M_Rad_links, P_Cl_V, P_Cl_Schlepp, P_Verz_V] = mUELG(M_Kupplung, M_Kupplung_mUELG_Schlepp, okay_CL, okay_CR, M_ein, M_RW, M_LW, n_ein, nri, nli, eta_Diff_mUELG, eta_Verz_mUELG, i_DF, z_ayc_lr, z_ayc_rl, z_atts, choose_ulg)
%berechnet das mechanische ÜLG
%M_RW, LW: Wunschmomente am linken sowie rechten Rad
%M_ein: Moment vom Getriebe
%nri: Ist-Drehzahl rechtes Rad
%nli: Ist-Drehzahl linkes Rad
%i_DF: Drehzahlfehlerübersetzung

%Initialisieren
M_D = M_ein*eta_Diff_mUELG/2;

%% Drehzahlfehler, Drehzahlen Kupplung, Grenzkurvenradius und Innen/Außendrehzahlen

% if nli > nri
%     na = nli;
%     ni = nri;
% else
%     na = nri;
%     ni = nli;
% end

%die vier Drehzahlen der Kupplungshälften:
%s1 ist stets die Scheibe, die angetrieben werden soll, d.h. die
%langsamere; erst unterhalb des GKR wird sie die schnellere

[ltr, rtl] = eval_Verlagerungsrichtung(M_RW, M_LW);

if ltr == 1
    z_ayc = z_ayc_lr;
elseif rtl == 1
    z_ayc = z_ayc_rl;
else
    z_ayc = 0;
end

switch choose_ulg
    case 0
        n_cl_s1 = nli;
        n_cl_s2 = nri/i_DF;
        n_cr_s1 = nri;
        n_cr_s2 = nli/i_DF;
    case 1
        n_cl_s1 = 0.5*(nli+nri)*z_ayc;
        n_cl_s2 = nri;
        n_cr_s1 = nri;
        n_cr_s2 = 0.5*(nri+nli)*z_ayc;
    case 2
        n_cl_s1 = nli*z_ayc;
        n_cl_s2 = nri;
        n_cr_s1 = nri;
        n_cr_s2 = nli*z_ayc;
    case 3
        n_cl_s1 = 0;
        n_cl_s2 = nri + 0.5*(nri-nli)*z_atts;
        n_cr_s1 = 0;
        n_cr_s2 = nli - 0.5*(nri-nli)*z_atts;
    otherwise
        n_cl_s1 = 0;
        n_cl_s2 = 0;
        n_cr_s1 = 0;
        n_cr_s2 = 0;
end

% DF = (1/i_DF-1)/(0.5*(1/i_DF+1));
% R_Grenz = s/DF;

%% Verlagerungslogik
switch choose_ulg
    case 0
        if rtl == 1
            M_Rad_rechts = M_D - M_Kupplung;
            M_Rad_links = M_D + M_Kupplung;
            if n_cl_s1 > n_cl_s2                    %unterhalb des GKR
                M_Rad_rechts = M_D + M_Kupplung;
                M_Rad_links = M_D - M_Kupplung;
            end
        elseif ltr == 1
            M_Rad_links = M_D - M_Kupplung; 
            M_Rad_rechts = M_D + M_Kupplung;
            if n_cr_s1 > n_cr_s2
                M_Rad_rechts = M_D - M_Kupplung;
                M_Rad_links = M_D + M_Kupplung;
            end
        else
            M_Rad_rechts = M_D;
            M_Rad_links = M_D;
        end
    case 1
         if rtl == 1
            M_Rad_rechts = M_D - M_Kupplung*(1-0.5*z_ayc_rl);
            M_Rad_links = M_D + M_Kupplung*0.5*z_ayc_rl;
            if n_cl_s1 > n_cl_s2                    %unterhalb des GKR
                M_Rad_rechts = M_D + M_Kupplung*0.5*z_ayc_rl;
                M_Rad_links = M_D - M_Kupplung*(1-0.5*z_ayc_rl);
            end
        elseif ltr == 1
            M_Rad_links = M_D - M_Kupplung*0.5*z_ayc_lr; 
            M_Rad_rechts = M_D + M_Kupplung*(1-0.5*z_ayc_lr);
            if n_cr_s1 > n_cr_s2
                M_Rad_rechts = M_D - M_Kupplung*0.5*z_ayc_lr;
                M_Rad_links = M_D + M_Kupplung*(1-0.5*z_ayc_lr);
        end
        else
            M_Rad_rechts = M_D;
            M_Rad_links = M_D;
         end
    case 2
         if rtl == 1
            M_Rad_rechts = M_D - M_Kupplung;
            M_Rad_links = M_D + M_Kupplung*z_ayc_rl;
            if n_cl_s1 > n_cl_s2                    %unterhalb des GKR
                M_Rad_rechts = M_D + M_Kupplung*z_ayc_rl;
                M_Rad_links = M_D - M_Kupplung;
            end
        elseif ltr == 1
            M_Rad_links = M_D - M_Kupplung*z_ayc_lr; 
            M_Rad_rechts = M_D + M_Kupplung;
            if n_cr_s1 > n_cr_s2
                M_Rad_rechts = M_D - M_Kupplung*z_ayc_lr;
                M_Rad_links = M_D + M_Kupplung;
            end
        else
            M_Rad_rechts = M_D;
            M_Rad_links = M_D;
         end
    case 3
         if rtl == 1
            M_Rad_rechts = M_D - M_Kupplung*(2+z_atts);
            M_Rad_links = M_D + M_Kupplung*z_atts;
            if n_cl_s1 > n_cl_s2                    %unterhalb des GKR
                M_Rad_rechts = M_D + M_Kupplung*z_atts;
                M_Rad_links = M_D - M_Kupplung*(2+z_atts);
            end
        elseif ltr == 1
            M_Rad_links = M_D - M_Kupplung*(2+z_atts); 
            M_Rad_rechts = M_D + M_Kupplung*z_atts;
            if n_cr_s1 > n_cr_s2
                M_Rad_rechts =M_D - M_Kupplung*(2+z_atts);
                M_Rad_links = M_D + M_Kupplung*z_atts;
            end
        else
            M_Rad_rechts = M_D;
            M_Rad_links = M_D;
         end
    otherwise
        M_Rad_rechts = M_D;
        M_Rad_links = M_D;
end

 
%Kupplungsverlustleistung (vorangegangener Zeitschritt)
P_Cl_V = 2*pi*M_Kupplung*(abs(n_cl_s1-n_cl_s2)*okay_CL + abs(n_cr_s1-n_cr_s2)*okay_CR);     %nur ein Term ist ungleich Null
P_Cl_Schlepp = 2*pi*M_Kupplung_mUELG_Schlepp*(abs(n_cl_s1-n_cl_s2)*okay_CL + abs(n_cr_s1-n_cr_s2)*okay_CR);
%Verlustleistung aus Verzahnung, MUSS VERFEINERT WERDEN
P_Verz_V = 2*pi*M_ein*n_ein*eta_Verz_mUELG*eta_Diff_mUELG;
end
